simulink model "cap"  (R2021b)
settings: Solver=FixedStepAuto  StartTime=0.0  StopTime=0.1  FixedStep=0.000001  RelTol=1e-3
libraries: spsDiodeLib x4, spsCurrentMeasurementLib x3, spsSeriesRLCBranchLib x3, spsVoltageMeasurementLib x2, spsACVoltageSourceLib x1, spsNeutralLib x1, spsVariableRatioTransformerLib x1, spspowerguiLib x1
settings Model: Creator=juheb  LastModifiedBy=juheb
settings DataIOCC: SaveFormat=Array  ReturnWorkspaceOutputs=off
settings HardwareCC: ProdBitPerLong=64  ProdLargestAtomicFloat=None  ProdHWDeviceType=AMD->Athlon 64

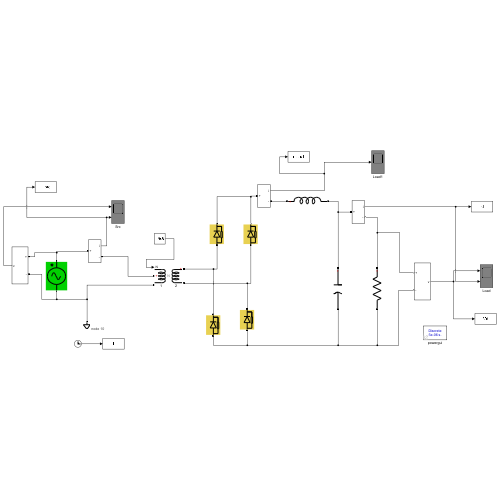
[thumbnail: Simulink's stored preview of the top-level diagram]
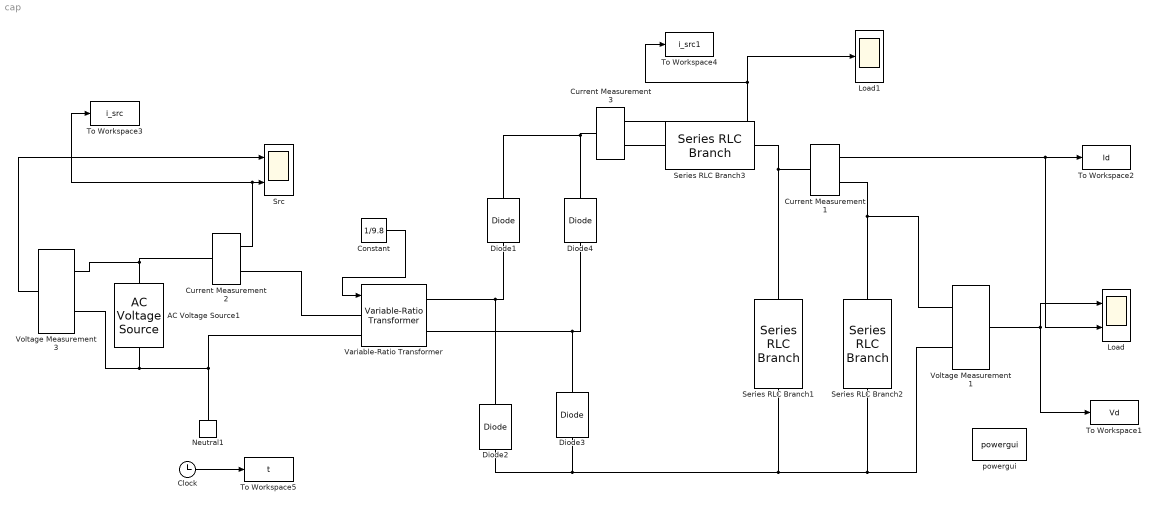
== system cap ==
  AC Voltage Source1 : spsACVoltageSourceLib/AC Voltage Source  Amplitude=230*sqrt(2)  Phase=0  Frequency=50  SampleTime=0  Measurements=None  BusType=swing  Pref=10e3  Qref=0  Qmin=-inf  Qmax=+inf
  Clock : Clock
  Constant : Constant  Value=1/9.8
  Current Measurement1 : spsCurrentMeasurementLib/Current Measurement  PhasorSimulation=off  OutputType=Complex  PSBequivalent=0
  Current Measurement2 : spsCurrentMeasurementLib/Current Measurement  PhasorSimulation=off  OutputType=Complex  PSBequivalent=0
  Current Measurement3 : spsCurrentMeasurementLib/Current Measurement  PhasorSimulation=off  OutputType=Complex  PSBequivalent=0
  Diode{1..4} (4 alike) : spsDiodeLib/Diode  Ron=0.001  Lon=0  Vf=0.8  IC=0  UseSnubber=off  Rs=500  Cs=250e-9  Measurements=off
  Load : Scope  NumInputPorts=2
  Load1 : Scope
  Neutral1 : spsNeutralLib/Neutral  LConnTagsString=a  NodeNumber=10
      settings: AttributesFormatString=node %<NodeNumber>  SourceProductBaseCode=PS
  Series RLC Branch1 : spsSeriesRLCBranchLib/Series RLC Branch  LConnTagsString=__new0  RConnTagsString=__new0  BranchType=C  Resistance=3  Inductance=0  SetiL0=off  InitialCurrent=0  Capacitance=0.0084  Setx0=off  InitialVoltage=0  Measurements=None
  Series RLC Branch2 : spsSeriesRLCBranchLib/Series RLC Branch  LConnTagsString=__new0  RConnTagsString=__new0  BranchType=R  Resistance=6  Inductance=0  SetiL0=off  InitialCurrent=0  Capacitance=0  Setx0=off  InitialVoltage=0  Measurements=None
  Series RLC Branch3 : spsSeriesRLCBranchLib/Series RLC Branch  LConnTagsString=__new0  RConnTagsString=__new0  BranchType=L  Resistance=3  Inductance=0.0009488  SetiL0=off  InitialCurrent=0  Capacitance=0.0084  Setx0=off  InitialVoltage=0  Measurements=None
  Src : Scope  NumInputPorts=2
  To Workspace1 : ToWorkspace  VariableName=Vd  SampleTime=-1
  To Workspace2 : ToWorkspace  VariableName=Id  SampleTime=-1
  To Workspace3 : ToWorkspace  VariableName=i_src  SampleTime=-1
  To Workspace4 : ToWorkspace  VariableName=i_src1  SampleTime=-1
  To Workspace5 : ToWorkspace  VariableName=t  SampleTime=-1
  Variable-Ratio Transformer : spsVariableRatioTransformerLib/Variable-Ratio Transformer
      settings: SourceProductBaseCode=PS
  Voltage Measurement1 : spsVoltageMeasurementLib/Voltage Measurement  PhasorSimulation=off  OutputType=Complex  PSBequivalent=0
  Voltage Measurement3 : spsVoltageMeasurementLib/Voltage Measurement  PhasorSimulation=off  OutputType=Complex  PSBequivalent=0
  powergui : spspowerguiLib/powergui  Priority=1  SimulationMode=Discrete  SampleTime=50e-7  frequency=60  Iterations=50  frequencyindice=50  Pbase=100e6  ErrMax=1e-4  UnitsV=kV  UnitsW=MW  buscounter=0  FunctionMessages=off  echomessages=off  EnableUseOfTLC=off  CurrentSourceSwitches=off  DisableSnubberDevices=off  DisableRonSwitches=off  DisableVfSwitches=off  DisplayEquations=off  AutomaticDiscreteSolvers=off  SolverType=Tustin  Interpol=off  ExternalGateDelay=off  methode=off  Ts=0  x0status=blocks  SPID=off  SwTol=0  HookPort=off  NonlinearTolerance=1e-4  nMaxIteration=100  ContinueOnMaxIteration=off  RestoreLinks=warning  ResistiveCurrentMeasurement=off  Frange=[0:2:500]  Ylog=off  Xlog=on  ShowGrid=off  save=off  variable=ZData  structure=0  ZoomFFT=off  StartTime=0.0  cycles=1  DisplayStyle=1  fundamental=60  FreqAxis=off  MaxFrequency=1000  frequencyindicesteady=1  RmsSteady=1  display=off
  wires:
  Current Measurement1/1 -> Load/2, To Workspace2/1
  Voltage Measurement1/1 -> Load/1, To Workspace1/1
  Voltage Measurement3/1 -> Src/1
  Clock/1 -> To Workspace5/1
  Current Measurement2/1 -> To Workspace3/1, Src/2
  Constant/1 -> Variable-Ratio Transformer/1
  Current Measurement3/1 -> To Workspace4/1, Load1/1
  connections:
  Diode3/LConn1 -- Diode2/LConn1 -- Series RLC Branch1/RConn1 -- Voltage Measurement1/LConn2 -- Series RLC Branch2/RConn1
  Voltage Measurement3/LConn2 -- Neutral1/LConn1 -- Variable-Ratio Transformer/LConn2 -- AC Voltage Source1/LConn1
  Current Measurement3/LConn1 -- Diode1/RConn1 -- Diode4/RConn1
  Current Measurement2/LConn1 -- AC Voltage Source1/RConn1 -- Voltage Measurement3/LConn1
  Series RLC Branch2/LConn1 -- Current Measurement1/RConn1 -- Voltage Measurement1/LConn1
  Variable-Ratio Transformer/RConn1 -- Diode1/LConn1 -- Diode2/RConn1
  Diode4/LConn1 -- Variable-Ratio Transformer/RConn2 -- Diode3/RConn1
  Variable-Ratio Transformer/LConn1 -- Current Measurement2/RConn1
  Series RLC Branch1/LConn1 -- Series RLC Branch3/RConn1 -- Current Measurement1/LConn1
  Current Measurement3/RConn1 -- Series RLC Branch3/LConn1
